simulink model "Gain_TestGen30"  (R2017b)
settings: Solver=FixedStepDiscrete  StartTime=0.0  StopTime=10.0  RelTol=1e-3
settings Model: Creator=ktrinh  LastModifiedBy=ktrinh
settings DebuggingCC: ParameterOverflowMsg=none

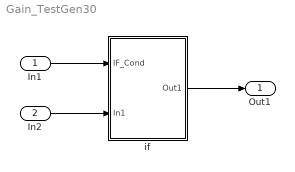
== system Gain_TestGen30 ==
  In1 : Inport
  In2 : Inport  Port=2
  if : Subsystem  AncestorBlock=Block_TestLib/if
  Out1 : Outport
  wires:
  In1/1 -> if/1(IF_Cond)
  In2/1 -> if/2(In1)
  if/1(Out1) -> Out1/1

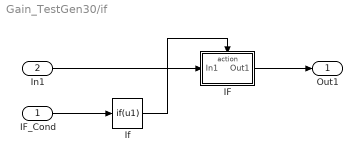
== system Gain_TestGen30/if ==
  IF_Cond : Inport  OutDataTypeStr=boolean
  In1 : Inport  Port=2
  IF : Subsystem  TreatAsAtomicUnit=on
  If : If  IfExpression=u1  ShowElse=off
  Out1 : Outport
  wires:
  If/1 -> IF/Action
  In1/1 -> IF/1(In1)
  IF_Cond/1 -> If/1
  IF/1(Out1) -> Out1/1

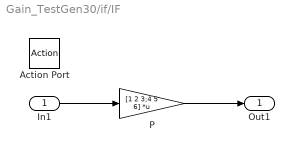
== system Gain_TestGen30/if/IF ==
  In1 : Inport  PortDimensions=[3,2]
  Action Port : ActionPort  ActionType=then
  P : Gain  Gain=[1 2 3;4 5 6]  Multiplication=Matrix(K*u)  ParamDataTypeStr=uint32  OutMin=1.  OutMax=100  OutDataTypeStr=uint32  RndMeth=Convergent  SaturateOnIntegerOverflow=on  LockScale=on
  Out1 : Outport
  wires:
  In1/1 -> P/1
  P/1 -> Out1/1
